simulink model "CounterWithReset"  (R2022b)
settings: Solver=VariableStepAuto  StartTime=0.0  StopTime=10.0  FixedStep=1  MaxStep=1  RelTol=1  AbsTol=1
settings Model: Creator=Mo_7atem  LastModifiedBy=Mo_7atem

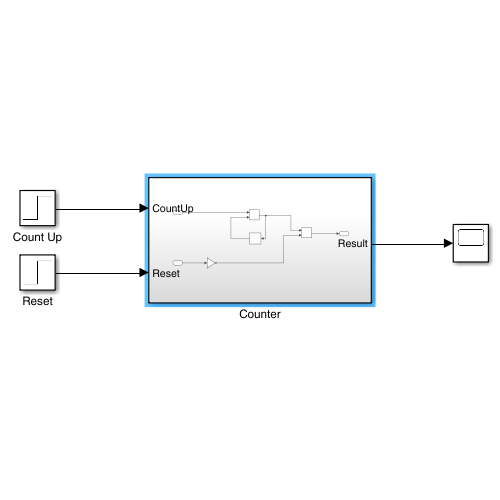
[thumbnail: Simulink's stored preview of the top-level diagram]
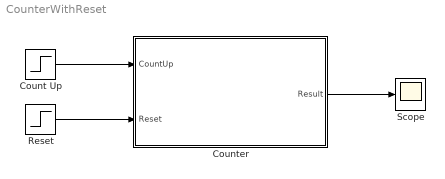
== system CounterWithReset ==
  Count Up : Step  SampleTime=0
  Counter : Subsystem
  Reset : Step  Time=5  SampleTime=0
  Scope : Scope
  wires:
  Count Up/1 -> Counter/1(CountUp)
  Reset/1 -> Counter/2(Reset)
  Counter/1(Result) -> Scope/1

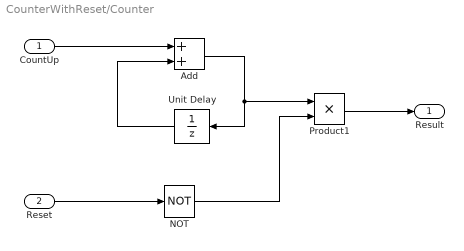
== system CounterWithReset/Counter ==
  CountUp : Inport
  Reset : Inport  Port=2
  Add : Sum
  NOT : Logic  Operator=NOT  IconShape=distinctive  AllPortsSameDT=off  OutDataTypeStr=boolean
  Product1 : Product
  Unit Delay : UnitDelay  SampleTime=-1  HasFrameUpgradeWarning=on
  Result : Outport
  wires:
  Unit Delay/1 -> Add/2
  Add/1 -> Product1/1, Unit Delay/1
  CountUp/1 -> Add/1
  Reset/1 -> NOT/1
  NOT/1 -> Product1/2
  Product1/1 -> Result/1
